simulink model "RandomResponseExperiment_SingleTank_2016a"  (R2017b)
settings: Solver=ode4  StartTime=0.0  StopTime=200  FixedStep=0.05  RelTol=1e-3
settings Model: Creator=HTH  LastModifiedBy=phamt
settings OptimizationCC: LifeSpan=inf
settings DebuggingCC: SFExecutionAtInitializationDiag=none
settings CodeAppCC: StateflowObjectComments=on

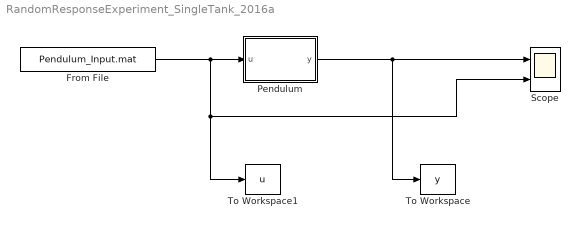
== system RandomResponseExperiment_SingleTank_2016a ==
  From File : FromFile  FileName=Pendulum_Input.mat
  Pendulum : Subsystem  mask{m=0.3, l=0.5, b=0.2, g=9.81}
  Scope : Scope  NumInputPorts=2
  To Workspace : ToWorkspace  VariableName=y  SampleTime=-1
  To Workspace1 : ToWorkspace  VariableName=u  SampleTime=-1
  wires:
  From File/1 -> Pendulum/1(u), Scope/2, To Workspace1/1
  Pendulum/1(y) -> To Workspace/1, Scope/1

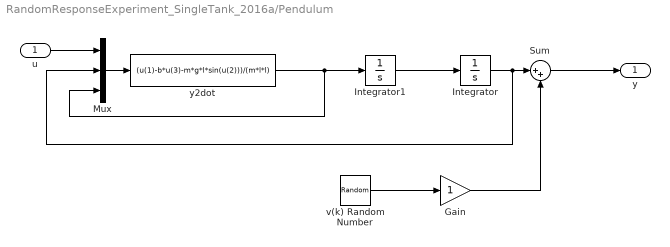
== system RandomResponseExperiment_SingleTank_2016a/Pendulum ==
  u : Inport
  Gain : Gain
  Integrator : Integrator  UpperSaturationLimit=pi/3  LowerSaturationLimit=-pi/3
  Integrator1 : Integrator  UpperSaturationLimit=pi/3  LowerSaturationLimit=-pi/3
  Mux : Mux  Inputs=3
  Sum : Sum  Inputs=|++
  v(k) Random Number : RandomNumber  Variance=0.001
  y2dot : Fcn  Expr=(u(1)-b*u(3)-m*g*l*sin(u(2)))/(m*l*l)
  y : Outport
  wires:
  Integrator/1 -> Mux/2, Sum/1
  y2dot/1 -> Mux/3, Integrator1/1
  Mux/1 -> y2dot/1
  u/1 -> Mux/1
  Sum/1 -> y/1
  v(k) Random Number/1 -> Gain/1
  Gain/1 -> Sum/2
  Integrator1/1 -> Integrator/1
